simulink model "CAN_TX_RX"  (R2020a)
settings: Solver=FixedStepDiscrete  StartTime=0.0  StopTime=10.0  FixedStep=50e-3  RelTol=1e-3  EnableMultiTasking=on
InitFcn:
  | mbd_s32k_consistency_checks(bdroot(gcs));
undefined symbols (not defined in the file or in its folder): Data, LQFP
libraries: mbd_s32k1xx_ec_toolbox x40, simulink x17, etargetslib x15
(part 2 of 2)

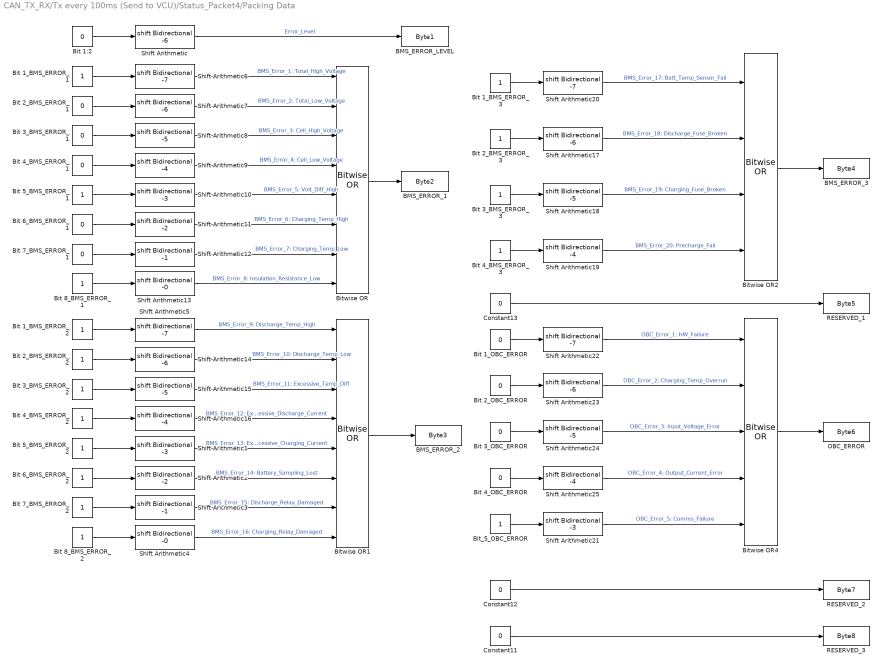
== system CAN_TX_RX/Tx every 100ms (Send to VCU)/Status_Packet4/Packing Data ==
  BMS_ERROR_1 : DataStoreWrite  DataStoreName=Byte2
  BMS_ERROR_2 : DataStoreWrite  DataStoreName=Byte3
  BMS_ERROR_3 : DataStoreWrite  DataStoreName=Byte4
  BMS_ERROR_LEVEL : DataStoreWrite  DataStoreName=Byte1
  Bit 1:2 : Constant  Value=0  OutDataTypeStr=uint8
  Bit 1_BMS_ERROR_1 : Constant  OutDataTypeStr=uint8
  Bit 1_BMS_ERROR_2 : Constant  OutDataTypeStr=uint8
  Bit 1_BMS_ERROR_3 : Constant  OutDataTypeStr=uint8
  Bit 1_OBC_ERROR : Constant  Value=0  OutDataTypeStr=uint8
  Bit 2_BMS_ERROR_1 : Constant  Value=0  OutDataTypeStr=uint8
  Bit 2_BMS_ERROR_2 : Constant  OutDataTypeStr=uint8
  Bit 2_BMS_ERROR_3 : Constant  OutDataTypeStr=uint8
  Bit 2_OBC_ERROR : Constant  Value=0  OutDataTypeStr=uint8
  Bit 3_BMS_ERROR_1 : Constant  Value=0  OutDataTypeStr=uint8
  Bit 3_BMS_ERROR_2 : Constant  OutDataTypeStr=uint8
  Bit 3_BMS_ERROR_3 : Constant  OutDataTypeStr=uint8
  Bit 3_OBC_ERROR : Constant  Value=0  OutDataTypeStr=uint8
  Bit 4_BMS_ERROR_1 : Constant  Value=0  OutDataTypeStr=uint8
  Bit 4_BMS_ERROR_2 : Constant  OutDataTypeStr=uint8
  Bit 4_BMS_ERROR_3 : Constant  OutDataTypeStr=uint8
  Bit 4_OBC_ERROR : Constant  Value=0  OutDataTypeStr=uint8
  Bit 5_BMS_ERROR_1 : Constant  OutDataTypeStr=uint8
  Bit 5_BMS_ERROR_2 : Constant  OutDataTypeStr=uint8
  Bit 6_BMS_ERROR_1 : Constant  Value=0  OutDataTypeStr=uint8
  Bit 6_BMS_ERROR_2 : Constant  OutDataTypeStr=uint8
  Bit 7_BMS_ERROR_1 : Constant  Value=0  OutDataTypeStr=uint8
  Bit 7_BMS_ERROR_2 : Constant  OutDataTypeStr=uint8
  Bit 8_BMS_ERROR_1 : Constant  OutDataTypeStr=uint8
  Bit 8_BMS_ERROR_2 : Constant  OutDataTypeStr=uint8
  Bit_5_OBC_ERROR : Constant  OutDataTypeStr=uint8
  Bitwise OR : simulink/Logic and Bit Operations/Bitwise Operator  logicop=OR  UseBitMask=off  NumInputPorts=8  BitMask=bin2dec('11011001')  BitMaskRealWorld=Stored Integer
  Bitwise OR1 : simulink/Logic and Bit Operations/Bitwise Operator  logicop=OR  UseBitMask=off  NumInputPorts=8  BitMask=bin2dec('11011001')  BitMaskRealWorld=Stored Integer
  Bitwise OR2 : simulink/Logic and Bit Operations/Bitwise Operator  logicop=OR  UseBitMask=off  NumInputPorts=4  BitMask=bin2dec('11011001')  BitMaskRealWorld=Stored Integer
  Bitwise OR4 : simulink/Logic and Bit Operations/Bitwise Operator  logicop=OR  UseBitMask=off  NumInputPorts=5  BitMask=bin2dec('11011001')  BitMaskRealWorld=Stored Integer
  Constant11 : Constant  Value=0  OutDataTypeStr=uint8
  Constant12 : Constant  Value=0  OutDataTypeStr=uint8
  Constant13 : Constant  Value=0  OutDataTypeStr=uint8
  OBC_ERROR : DataStoreWrite  DataStoreName=Byte6
  RESERVED_1 : DataStoreWrite  DataStoreName=Byte5
  RESERVED_2 : DataStoreWrite  DataStoreName=Byte7
  RESERVED_3 : DataStoreWrite  DataStoreName=Byte8
  Shift Arithmetic{,7,14,17,23} (5 alike) : ArithShift  BitShiftNumber=-6
  Shift Arithmetic1 : ArithShift  BitShiftNumber=-3
  Shift Arithmetic10 : ArithShift  BitShiftNumber=-3
  Shift Arithmetic11 : ArithShift  BitShiftNumber=-2
  Shift Arithmetic12 : ArithShift  BitShiftNumber=-1
  Shift Arithmetic13 : ArithShift  BitShiftNumber=-0
  Shift Arithmetic{8,15,18,24} (4 alike) : ArithShift  BitShiftNumber=-5
  Shift Arithmetic{9,16,19,25} (4 alike) : ArithShift  BitShiftNumber=-4
  Shift Arithmetic2 : ArithShift  BitShiftNumber=-2
  Shift Arithmetic{5..6,20,22} (4 alike) : ArithShift  BitShiftNumber=-7
  Shift Arithmetic21 : ArithShift  BitShiftNumber=-3
  Shift Arithmetic3 : ArithShift  BitShiftNumber=-1
  Shift Arithmetic4 : ArithShift  BitShiftNumber=-0
  wires:
  Bit 1:2/1 -> Shift Arithmetic/1
  Constant11/1 -> RESERVED_3/1
  Constant12/1 -> RESERVED_2/1
  Constant13/1 -> RESERVED_1/1
  Shift Arithmetic/1 -> BMS_ERROR_LEVEL/1  "Error_Level"
  Bitwise OR/1 -> BMS_ERROR_1/1
  Shift Arithmetic6/1 -> Bitwise OR/1  "BMS_Error_1: Total_High_Voltage"
  Shift Arithmetic7/1 -> Bitwise OR/2  "BMS_Error_2: Total_Low_Voltage"
  Shift Arithmetic8/1 -> Bitwise OR/3  "BMS_Error_3: Cell_High_Voltage"
  Shift Arithmetic9/1 -> Bitwise OR/4  "BMS_Error_4: Cell_Low_Voltage"
  Shift Arithmetic10/1 -> Bitwise OR/5  "BMS_Error_5: Volt_Diff_High"
  Shift Arithmetic11/1 -> Bitwise OR/6  "BMS_Error_6: Charging_Temp_High"
  Shift Arithmetic12/1 -> Bitwise OR/7  "BMS_Error_7: Charging_Temp_Low"
  Shift Arithmetic13/1 -> Bitwise OR/8  "BMS_Error_8: Insulation_Resistance_Low"
  Bit 1_BMS_ERROR_1/1 -> Shift Arithmetic6/1
  Bit 2_BMS_ERROR_1/1 -> Shift Arithmetic7/1
  Bit 3_BMS_ERROR_1/1 -> Shift Arithmetic8/1
  Bit 4_BMS_ERROR_1/1 -> Shift Arithmetic9/1
  Bit 5_BMS_ERROR_1/1 -> Shift Arithmetic10/1
  Bit 6_BMS_ERROR_1/1 -> Shift Arithmetic11/1
  Bit 7_BMS_ERROR_1/1 -> Shift Arithmetic12/1
  Bit 8_BMS_ERROR_1/1 -> Shift Arithmetic13/1
  Bitwise OR1/1 -> BMS_ERROR_2/1
  Shift Arithmetic5/1 -> Bitwise OR1/1  "BMS_Error_9: Discharge_Temp_High"
  Shift Arithmetic14/1 -> Bitwise OR1/2  "BMS_Error_10: Discharge_Temp_Low"
  Shift Arithmetic15/1 -> Bitwise OR1/3  "BMS_Error_11: Excessive_Temp_Diff"
  Shift Arithmetic16/1 -> Bitwise OR1/4  "BMS_Error_12: Excessive_Discharge_Current"
  Shift Arithmetic1/1 -> Bitwise OR1/5  "BMS_Error_13: Excessive_Charging_Current"
  Shift Arithmetic2/1 -> Bitwise OR1/6  "BMS_Error_14: Battery_Sampling_Lost"
  Shift Arithmetic3/1 -> Bitwise OR1/7  "BMS_Error_15: Discharge_Relay_Damaged"
  Shift Arithmetic4/1 -> Bitwise OR1/8  "BMS_Error_16: Charging_Relay_Damaged"
  Bit 1_BMS_ERROR_2/1 -> Shift Arithmetic5/1
  Bit 2_BMS_ERROR_2/1 -> Shift Arithmetic14/1
  Bit 3_BMS_ERROR_2/1 -> Shift Arithmetic15/1
  Bit 4_BMS_ERROR_2/1 -> Shift Arithmetic16/1
  Bit 5_BMS_ERROR_2/1 -> Shift Arithmetic1/1
  Bit 6_BMS_ERROR_2/1 -> Shift Arithmetic2/1
  Bit 7_BMS_ERROR_2/1 -> Shift Arithmetic3/1
  Bit 8_BMS_ERROR_2/1 -> Shift Arithmetic4/1
  Bitwise OR2/1 -> BMS_ERROR_3/1
  Shift Arithmetic20/1 -> Bitwise OR2/1  "BMS_Error_17: Batt_Temp_Sensor_Fail"
  Shift Arithmetic19/1 -> Bitwise OR2/4  "BMS_Error_20: Precharge_Fail"
  Shift Arithmetic18/1 -> Bitwise OR2/3  "BMS_Error_19: Charging_Fuse_Broken"
  Shift Arithmetic17/1 -> Bitwise OR2/2  "BMS_Error_18: Discharge_Fuse_Broken"
  Bit 1_BMS_ERROR_3/1 -> Shift Arithmetic20/1
  Bit 2_BMS_ERROR_3/1 -> Shift Arithmetic17/1
  Bit 3_BMS_ERROR_3/1 -> Shift Arithmetic18/1
  Bit 4_BMS_ERROR_3/1 -> Shift Arithmetic19/1
  Bitwise OR4/1 -> OBC_ERROR/1
  Shift Arithmetic21/1 -> Bitwise OR4/5  "OBC_Error_5: Comms_Failure"
  Shift Arithmetic25/1 -> Bitwise OR4/4  "OBC_Error_4: Output_Current_Error"
  Shift Arithmetic24/1 -> Bitwise OR4/3  "OBC_Error_3: Input_Voltage_Error"
  Shift Arithmetic23/1 -> Bitwise OR4/2  "OBC_Error_2: Charging_Temp_Overrun"
  Shift Arithmetic22/1 -> Bitwise OR4/1  "OBC_Error_1: HW_Failure"
  Bit 1_OBC_ERROR/1 -> Shift Arithmetic22/1
  Bit 2_OBC_ERROR/1 -> Shift Arithmetic23/1
  Bit 3_OBC_ERROR/1 -> Shift Arithmetic24/1
  Bit 4_OBC_ERROR/1 -> Shift Arithmetic25/1
  Bit_5_OBC_ERROR/1 -> Shift Arithmetic21/1

== system CAN_TX_RX/Tx every 200ms (Send to VCU)/Status_Packet2/Grouping Data ==
  Byte Pack1 : etargetslib/Byte Pack  datatypes={'uint16', 'uint16', 'uint16', 'uint16'}  byteAlign=1
  Data Store Read6 : DataStoreRead  DataStoreName=Byte1_2
  Data Store Read7 : DataStoreRead  DataStoreName=Byte3_4
  Data Store Read8 : DataStoreRead  DataStoreName=Byte5_6
  Data Store Read9 : DataStoreRead  DataStoreName=Byte7_8
  Packet2 : Outport
  wires:
  Data Store Read6/1 -> Byte Pack1/1
  Data Store Read7/1 -> Byte Pack1/2
  Data Store Read8/1 -> Byte Pack1/3
  Data Store Read9/1 -> Byte Pack1/4
  Byte Pack1/1 -> Packet2/1

== system CAN_TX_RX/Tx every 200ms (Send to VCU)/Status_Packet2/Packing Data ==
  Constant : Constant  Value=5000  OutDataTypeStr=uint16
  Constant1 : Constant  Value=4000  OutDataTypeStr=uint16
  Constant2 : Constant  Value=800  OutDataTypeStr=uint16
  Constant3 : Constant  Value=640  OutDataTypeStr=uint16
  HIGHEST_CELL_VOLTAGE : DataStoreWrite  DataStoreName=Byte5_6
  LOWEST_CELL_VOLTAGE : DataStoreWrite  DataStoreName=Byte7_8
  MAX_BUS_CURRENT : DataStoreWrite  DataStoreName=Byte1_2
  MAX_REGEN_CURRENT : DataStoreWrite  DataStoreName=Byte3_4
  wires:
  Constant/1 -> MAX_BUS_CURRENT/1
  Constant1/1 -> MAX_REGEN_CURRENT/1
  Constant2/1 -> HIGHEST_CELL_VOLTAGE/1
  Constant3/1 -> LOWEST_CELL_VOLTAGE/1

== system CAN_TX_RX/Tx every 200ms (Send to VCU)/Status_Packet3/Grouping Data ==
  Byte Pack : etargetslib/Byte Pack  datatypes={'uint16'}  byteAlign=1
  Data Store Read10 : DataStoreRead  DataStoreName=Byte4
  Data Store Read4 : DataStoreRead  DataStoreName=Byte5_6
  Data Store Read5 : DataStoreRead  DataStoreName=Byte7
  Data Store Read6 : DataStoreRead  DataStoreName=Byte8
  Data Store Read7 : DataStoreRead  DataStoreName=Byte1
  Data Store Read8 : DataStoreRead  DataStoreName=Byte2
  Data Store Read9 : DataStoreRead  DataStoreName=Byte3
  Mux : Mux  Inputs=7
  Packet3 : Outport
  wires:
  Mux/1 -> Packet3/1
  Data Store Read4/1 -> Byte Pack/1
  Data Store Read7/1 -> Mux/1
  Data Store Read8/1 -> Mux/2
  Data Store Read10/1 -> Mux/4
  Data Store Read9/1 -> Mux/3
  Data Store Read5/1 -> Mux/6
  Data Store Read6/1 -> Mux/7
  Byte Pack/1 -> Mux/5

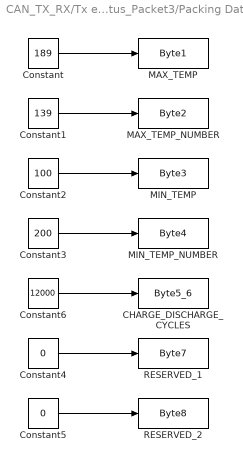
== system CAN_TX_RX/Tx every 200ms (Send to VCU)/Status_Packet3/Packing Data ==
  CHARGE_DISCHARGE_CYCLES : DataStoreWrite  DataStoreName=Byte5_6
  Constant : Constant  Value=189  OutDataTypeStr=uint8
  Constant1 : Constant  Value=139  OutDataTypeStr=uint8
  Constant2 : Constant  Value=100  OutDataTypeStr=uint8
  Constant3 : Constant  Value=200  OutDataTypeStr=uint8
  Constant4 : Constant  Value=0  OutDataTypeStr=uint8
  Constant5 : Constant  Value=0  OutDataTypeStr=uint8
  Constant6 : Constant  Value=12000  OutDataTypeStr=uint16
  MAX_TEMP : DataStoreWrite  DataStoreName=Byte1
  MAX_TEMP_NUMBER : DataStoreWrite  DataStoreName=Byte2
  MIN_TEMP : DataStoreWrite  DataStoreName=Byte3
  MIN_TEMP_NUMBER : DataStoreWrite  DataStoreName=Byte4
  RESERVED_1 : DataStoreWrite  DataStoreName=Byte7
  RESERVED_2 : DataStoreWrite  DataStoreName=Byte8
  wires:
  Constant4/1 -> RESERVED_1/1
  Constant5/1 -> RESERVED_2/1
  Constant6/1 -> CHARGE_DISCHARGE_CYCLES/1
  Constant3/1 -> MIN_TEMP_NUMBER/1
  Constant2/1 -> MIN_TEMP/1
  Constant/1 -> MAX_TEMP/1
  Constant1/1 -> MAX_TEMP_NUMBER/1

== system CAN_TX_RX/Tx every 50ms (Send to VCU)/Status_Packet1/Grouping Data ==
  Byte Pack : etargetslib/Byte Pack  datatypes={'uint16', 'uint16'}  byteAlign=1
  Data Store Read : DataStoreRead  DataStoreName=Byte1
  Data Store Read1 : DataStoreRead  DataStoreName=Byte2
  Data Store Read2 : DataStoreRead  DataStoreName=Byte3
  Data Store Read3 : DataStoreRead  DataStoreName=Byte4_5
  Data Store Read4 : DataStoreRead  DataStoreName=Byte6_7
  Data Store Read5 : DataStoreRead  DataStoreName=Byte8
  Mux : Mux  Inputs=5
  Packet1 : Outport
  wires:
  Data Store Read4/1 -> Byte Pack/2
  Data Store Read1/1 -> Mux/2
  Byte Pack/1 -> Mux/4
  Data Store Read5/1 -> Mux/5
  Data Store Read3/1 -> Byte Pack/1
  Data Store Read/1 -> Mux/1
  Data Store Read2/1 -> Mux/3
  Mux/1 -> Packet1/1

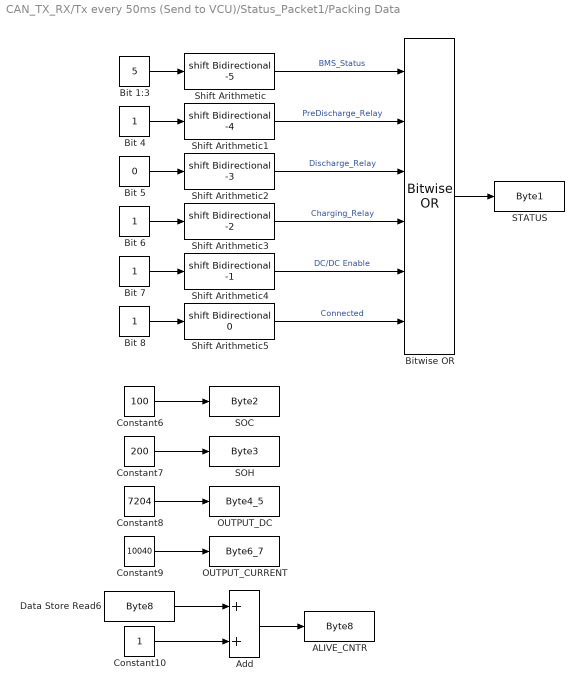
== system CAN_TX_RX/Tx every 50ms (Send to VCU)/Status_Packet1/Packing Data ==
  ALIVE_CNTR : DataStoreWrite  DataStoreName=Byte8
  Add : Sum
  Bit 1:3 : Constant  Value=5  OutDataTypeStr=uint8
  Bit {4,6..8} (4 alike) : Constant  OutDataTypeStr=uint8
  Bit 5 : Constant  Value=0  OutDataTypeStr=uint8
  Bitwise OR : simulink/Logic and Bit Operations/Bitwise Operator  logicop=OR  UseBitMask=off  NumInputPorts=6  BitMask=bin2dec('11011001')  BitMaskRealWorld=Stored Integer
  Constant10 : Constant  OutDataTypeStr=uint8
  Constant6 : Constant  Value=100  OutDataTypeStr=uint8
  Constant7 : Constant  Value=200  OutDataTypeStr=uint8
  Constant8 : Constant  Value=7204  OutDataTypeStr=uint16
  Constant9 : Constant  Value=10040  OutDataTypeStr=uint16
  Data Store Read6 : DataStoreRead  DataStoreName=Byte8
  OUTPUT_CURRENT : DataStoreWrite  DataStoreName=Byte6_7
  OUTPUT_DC : DataStoreWrite  DataStoreName=Byte4_5
  SOC : DataStoreWrite  DataStoreName=Byte2
  SOH : DataStoreWrite  DataStoreName=Byte3
  STATUS : DataStoreWrite  DataStoreName=Byte1
  Shift Arithmetic : ArithShift  BitShiftNumber=-5
  Shift Arithmetic1 : ArithShift  BitShiftNumber=-4
  Shift Arithmetic2 : ArithShift  BitShiftNumber=-3
  Shift Arithmetic3 : ArithShift  BitShiftNumber=-2
  Shift Arithmetic4 : ArithShift  BitShiftNumber=-1
  Shift Arithmetic5 : ArithShift
  wires:
  Constant9/1 -> OUTPUT_CURRENT/1
  Shift Arithmetic1/1 -> Bitwise OR/2  "PreDischarge_Relay"
  Data Store Read6/1 -> Add/1
  Constant7/1 -> SOH/1
  Bitwise OR/1 -> STATUS/1
  Constant10/1 -> Add/2
  Shift Arithmetic3/1 -> Bitwise OR/4  "Charging_Relay"
  Shift Arithmetic2/1 -> Bitwise OR/3  "Discharge_Relay"
  Constant8/1 -> OUTPUT_DC/1
  Bit 5/1 -> Shift Arithmetic2/1
  Constant6/1 -> SOC/1
  Shift Arithmetic4/1 -> Bitwise OR/5  "DC/DC Enable"
  Bit 8/1 -> Shift Arithmetic5/1
  Bit 6/1 -> Shift Arithmetic3/1
  Bit 4/1 -> Shift Arithmetic1/1
  Shift Arithmetic5/1 -> Bitwise OR/6  "Connected"
  Shift Arithmetic/1 -> Bitwise OR/1  "BMS_Status"
  Bit 1:3/1 -> Shift Arithmetic/1
  Bit 7/1 -> Shift Arithmetic4/1
  Add/1 -> ALIVE_CNTR/1
